simulink library "OutCommunication"  (R2016b)
settings: Solver=VariableStepAuto  StartTime=0.0  StopTime=10.0  RelTol=1e-3
libraries: SendToSOMANET x8, VariousLibrary x2, SendToInputDevice x2, SendToPDB x2
settings Model: Creator=Nathan  LastModifiedBy=march

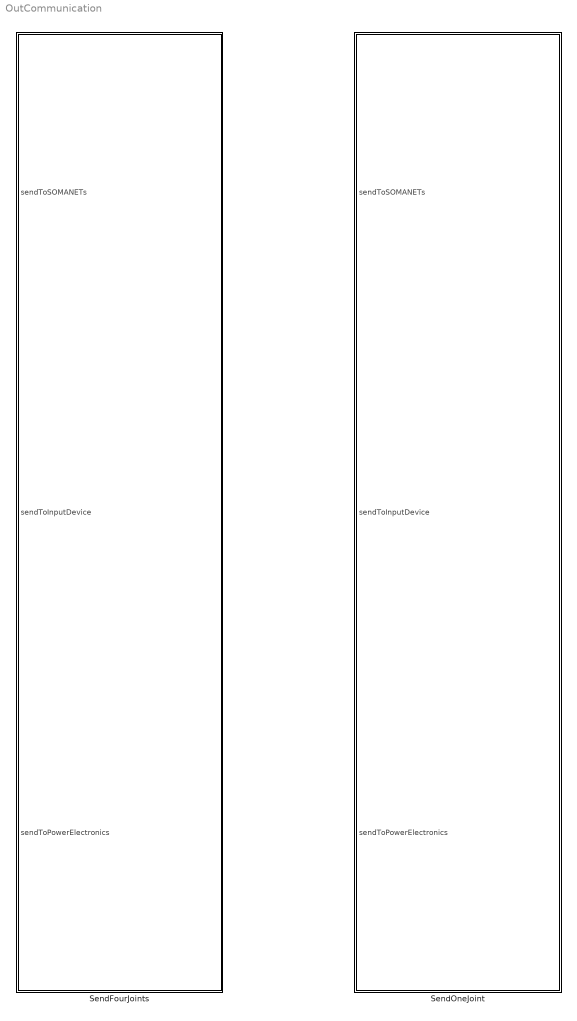
== system OutCommunication ==
  SendFourJoints : Subsystem
  SendOneJoint : Subsystem

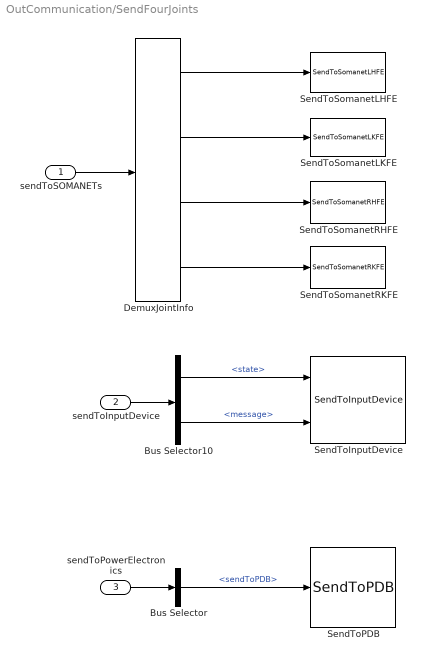
== system OutCommunication/SendFourJoints ==
  sendToSOMANETs : Inport  OutDataTypeStr=Bus: EtherCATSendToSOMANET  PortDimensions=[1 4]  BusOutputAsStruct=on
  sendToInputDevice : Inport  Port=2  OutDataTypeStr=Bus: EtherCATSendToInputDevice  BusOutputAsStruct=on
  sendToPowerElectronics : Inport  Port=3  OutDataTypeStr=Bus: EtherCATSendToPowerElectronics  BusOutputAsStruct=on
  Bus Selector : BusSelector  OutputSignals=sendToPDB
  Bus Selector10 : BusSelector  OutputSignals=state,message
  DemuxJointInfo : VariousLibrary/DemuxJointInfo
  SendToInputDevice : SendToInputDevice/SendToInputDevice
  SendToPDB : SendToPDB/SendToPDB
  SendToSomanetLHFE : SendToSOMANET/SendToSomanetLHFE
  SendToSomanetLKFE : SendToSOMANET/SendToSomanetLKFE
  SendToSomanetRHFE : SendToSOMANET/SendToSomanetRHFE
  SendToSomanetRKFE : SendToSOMANET/SendToSomanetRKFE
  wires:
  Bus Selector/1 -> SendToPDB/1  "<sendToPDB>"
  sendToSOMANETs/1 -> DemuxJointInfo/1
  DemuxJointInfo/3 -> SendToSomanetRHFE/1
  DemuxJointInfo/2 -> SendToSomanetLKFE/1
  DemuxJointInfo/1 -> SendToSomanetLHFE/1
  Bus Selector10/2 -> SendToInputDevice/2  "<message>"
  sendToPowerElectronics/1 -> Bus Selector/1
  Bus Selector10/1 -> SendToInputDevice/1  "<state>"
  DemuxJointInfo/4 -> SendToSomanetRKFE/1
  sendToInputDevice/1 -> Bus Selector10/1

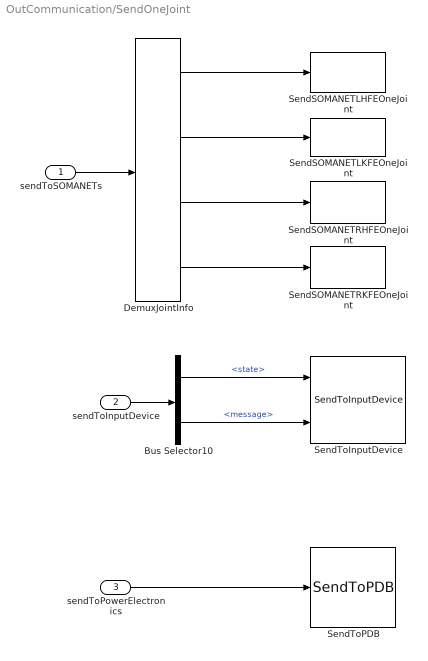
== system OutCommunication/SendOneJoint ==
  sendToSOMANETs : Inport  OutDataTypeStr=Bus: EtherCATSendToSOMANET  PortDimensions=[1 4]  BusOutputAsStruct=on
  sendToInputDevice : Inport  Port=2  OutDataTypeStr=Bus: EtherCATSendToInputDevice  BusOutputAsStruct=on
  sendToPowerElectronics : Inport  Port=3  OutDataTypeStr=Bus: EtherCATSendToPDB  BusOutputAsStruct=on
  Bus Selector10 : BusSelector  OutputSignals=state,message
  DemuxJointInfo : VariousLibrary/DemuxJointInfo
  SendSOMANETLHFEOneJoint : SendToSOMANET/SendSOMANETLHFEOneJoint
  SendSOMANETLKFEOneJoint : SendToSOMANET/SendSOMANETLKFEOneJoint
  SendSOMANETRHFEOneJoint : SendToSOMANET/SendSOMANETRHFEOneJoint
  SendSOMANETRKFEOneJoint : SendToSOMANET/SendSOMANETRKFEOneJoint
  SendToInputDevice : SendToInputDevice/SendToInputDevice
  SendToPDB : SendToPDB/SendToPDB
  wires:
  sendToInputDevice/1 -> Bus Selector10/1
  DemuxJointInfo/4 -> SendSOMANETRKFEOneJoint/1
  Bus Selector10/1 -> SendToInputDevice/1  "<state>"
  sendToPowerElectronics/1 -> SendToPDB/1
  Bus Selector10/2 -> SendToInputDevice/2  "<message>"
  DemuxJointInfo/1 -> SendSOMANETLHFEOneJoint/1
  DemuxJointInfo/2 -> SendSOMANETLKFEOneJoint/1
  DemuxJointInfo/3 -> SendSOMANETRHFEOneJoint/1
  sendToSOMANETs/1 -> DemuxJointInfo/1
